simulink model "HEVPlant_Ptbs_V1b_MkSfunc"  (R2018b)
settings: configuration reference "Config_Plant_MkSfunc_FIxStep" (kept outside this file)
PreLoadFcn:
  | HEVPlant_Ptbs_V1_BusInfo
model workspace (MAT data in the model file):
  DiffRatio = 3.421
  EV_current = 200
  EV_motion = [20 4 0.8]
  EV_sf = 2000
  EngDriveRatio = 0.813008130081
  Fs = 0
  Fv = 0.0025
  Jcomp = 0.0227
  Jengine = 0.22
  Ki = 251.3274
  Kisa = 346.6583
  Kp_d = 0.47149
  Kp_q = 0.52125
  Ksa = 85.4316
  Ksf = 1996.2651
  Ld = 0.0003752
  Ldq = [0.0003752 0.0004148]
  Lq = 0.0004148
  Mechanical = [0.0227 0.0025 0]
  MotGbRatio = 1
  P = 4
  PolePairs = 4
  RWheel = 0.3
  Rs = 0.2
  T_max = 120
  T_mtpa = [0 13.3131834767 26.6278836885 39.9456159322 53.2678926341 66.5962219318 79.9321062746 93.277041051 106.632513247 120.000000141]
  MCOS : class17 (value not decoded)
  MCOS : class17 (value not decoded)
  ba = 3.4029
  id_mtpa = [0 -0.114523352646 -0.457989076459 -1.03008464374 -1.83029075221 -2.85788367342 -4.11193850568 -5.59133329791 -7.29475400168 -9.22070020138]
  idq0 = [0 0]
  idq_limits = [-9.220699542 166.993501392 167.247872355]
  iq_mtpa = [0 18.5827440345 37.1633719111 55.7397734896 74.3098506185 92.871523015 111.422734008 129.961456105 148.485696337 166.993501356]
  MCOS : class17 (value not decoded)
  MCOS : class17 (value not decoded)
  lambda_pm = 0.1194
  mechanical = [0.0227 0.0025 0]
  mot : struct (value not decoded)
  omega_init = 0
  theta_init = 0
  MCOS : class17 (value not decoded)
symbols that are objects in the model workspace (value not decoded): mot
libraries: autolibshared x4, autolibsharedcoupling x2, autolibtransamt x1, autolibshareddiff x1, autolibsharedmappedengines x1, simulink x1, autolibdatasheetbattery x1, autolibmappedmotor x1
(part 5 of 5)

== system HEVPlant_Ptbs_V1b_MkSfunc/Engine/Info_in ==
  Bus Creator1 : BusCreator  Inputs=1
  Constant : Constant
  Info_in : Outport
  wires:
  Constant/1 -> Bus Creator1/1  "dummy"
  Bus Creator1/1 -> Info_in/1  "Info_in"

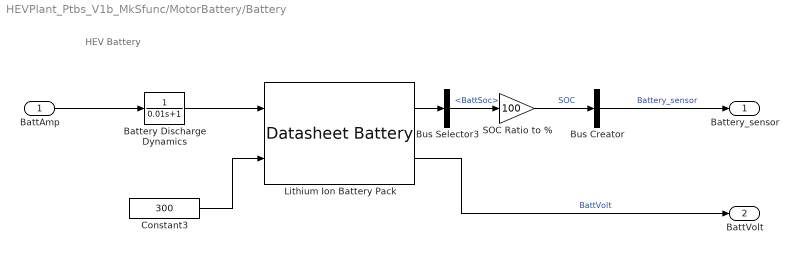
== system HEVPlant_Ptbs_V1b_MkSfunc/MotorBattery/Battery ==
  note: HEV Battery
  BattAmp : Inport
  Battery Discharge Dynamics : TransferFcn  Denominator=[0.01 1]
  Bus Creator : BusCreator  Inputs=1  OutDataTypeStr=Bus: Battery_sensor_Bus
      settings: AttributesFormatString=%<OutDataTypeStr>
  Bus Selector3 : BusSelector  OutputSignals=BattSoc
  Constant3 : Constant  Value=300
  Lithium Ion Battery Pack : autolibdatasheetbattery/Datasheet Battery  CapacityCtrl=Parameter  OutputVlt=Unfiltered  BattChargeMax=7  Em=[2.8 3.228 3.284 3.361 3.408 3.427 3.472 3.477 3.493 3.504 3.516 3.528 3.537 3.545 3.555 3.561 3.566 3.576 3.587 3.589 3.594 3.6 3.608 3.61 3.616 3.619 3.626 3.632 3.637 3.64 3.645 3.646 3.652 3.655 3.658 3.661 3.664 3.668 3.673 3.678 3.68 3.681 3.686 3.692 3.699 3.702 3.705 3.71 3.717 3.723 3.728 3.733 3.735 3.742 3.749 3.755 3.761 3.768 3.773 3.78 3.791 3.798 3.798 3.814 3.818 3.825 3.841 3.846 3.855 3.863 3.877 3.885 3.894 3.907 3.919 3.926 3.935 3.944 3.954 3.964 3.974 3.988 3.998 4.014 4.029 4.034 4.047 4.065 4.074 4.086 4.097 4.131 4.126 4.138 4.15 4.18 4.174 4.187 4.207 4.231 4.221]  CapLUTBp=[0 0.01 0.02 0.03 0.04 0.05 0.06 0.07 0.08 0.09 0.1 0.11 0.12 0.13 0.14 0.15 0.16 0.17 0.18 0.19 0.2 0.21 0.22 0.23 0.24 0.25 0.26 0.27 0.28 0.29 0.3 0.31 0.32 0.33 0.34 0.35 0.36 0.37 0.38 0.39 0.4 0.41 0.42 0.43 0.44 0.45 0.46 0.47 0.48 0.49 0.5 0.51 0.52 0.53 0.54 0.55 0.56 0.57 0.58 0.59 0.6 0.61 0.62 0.63 0.64 0.65 0.66 0.67 0.68 0.69 0.7 0.71 0.72 0.73 0.74 0.75 0.76 0.77 0.78 0.79 0.8 0.81 0.82 0.83 0.84 0.85 0.86 0.87 0.88 0.89 0.9 0.91 0.92 0.93 0.94 0.95 0.96 0.97 0.98 0.99 1]  RInt=[0.008846 0.009319 0.009027 0.00847 0.01032 0.01314;0.006389 0.006554 0.005553 0.005525 0.006043 0.007805;0.004364 0.004101 0.00406 0.003452 0.003846 0.004517;0.002031 0.002563 0.002532 0.00246 0.002716 0.003047;0.001443 0.001825 0.001795 0.001778 0.001924 0.002234;0.0005603 0.0007192 0.0006887 0.0007557 0.0007355 0.001014;0.001028 0.001338 0.001 0.001536 0.001546 0.002789]  BattTempBp=[243.1 253.1 263.1 273.1 283.1 298.1 313.1]  CapSOCBp=[0 0.2 0.4 0.6 0.8 1]  Ns=320/4.2  Np=1  BattCapInit=7*.6  Tc=1/1000  Vinit=4.221
      settings: SourceProductName=Powertrain Blockset  SourceProductBaseCode=PW
  SOC Ratio to % : Gain  Gain=100
  Battery_sensor : Outport
  BattVolt : Outport  Port=2
  wires:
  SOC Ratio to %/1 -> Bus Creator/1  "SOC"
  Lithium Ion Battery Pack/1 -> Bus Selector3/1
  Bus Selector3/1 -> SOC Ratio to %/1  "<BattSoc>"
  Constant3/1 -> Lithium Ion Battery Pack/2
  Battery Discharge Dynamics/1 -> Lithium Ion Battery Pack/1
  Bus Creator/1 -> Battery_sensor/1  "Battery_sensor"
  Lithium Ion Battery Pack/2 -> BattVolt/1  "BattVolt"
  BattAmp/1 -> Battery Discharge Dynamics/1

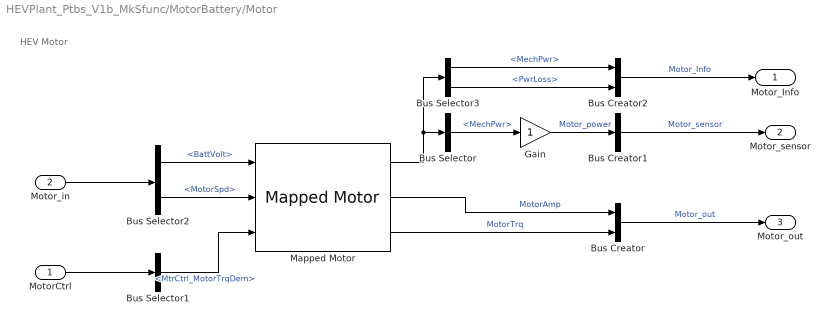
== system HEVPlant_Ptbs_V1b_MkSfunc/MotorBattery/Motor ==
  note: HEV Motor
  MotorCtrl : Inport  OutDataTypeStr=Bus: MotorCtrl_Bus  SampleTime=0
      settings: AttributesFormatString=%<OutDataTypeStr>
  Motor_in : Inport  Port=2  OutDataTypeStr=Bus: Motor_in_Bus
      settings: AttributesFormatString=%<OutDataTypeStr>
  Bus Creator : BusCreator  Inputs=2  OutDataTypeStr=Bus: Motor_out_Bus
      settings: AttributesFormatString=%<OutDataTypeStr>
  Bus Creator1 : BusCreator  Inputs=1  OutDataTypeStr=Bus: Motor_sensor_Bus
      settings: AttributesFormatString=%<OutDataTypeStr>
  Bus Creator2 : BusCreator  Inputs=2  OutDataTypeStr=Bus: Motor_Info_out_Bus
      settings: AttributesFormatString=%<OutDataTypeStr>
  Bus Selector : BusSelector  OutputSignals=MechPwr
  Bus Selector1 : BusSelector  OutputSignals=MtrCtrl_MotorTrqDem
  Bus Selector2 : BusSelector  OutputSignals=BattVolt,MotorSpd
  Bus Selector3 : BusSelector  OutputSignals=MechPwr,PwrLoss
  Gain : Gain
  Mapped Motor : autolibmappedmotor/Mapped Motor  port_config=Speed  param_by=Maximum torque and power  w_t=[ 0 375 750 800 ]  T_t=[0.09 0.08 0.07 0]  torque_max=307  power_max=124e3  Tc=0.02  param_loss=Tabulated efficiency data  eff=100  w_eff=375  T_eff=0.08  Piron=0  Pbase=0  w_eff_bp=mot.map.spdindex.*pi/30  T_eff_bp=mot.map.trqindex  losses_table=[1 2;3 4]  efficiency_table=mot.map.eff'  J=5e-6  b=1e-5  omega_o=0  T_t_extended=[0 0.07 0.08 0.09 0.08 0.07 0]  w_t_extended=[-800 -750 -375 0 375 750 800]  KLossIron=0  KLossCopper=0  x_w_eff_vec=[-1317.7933984258 -1256.63706143592 -1151.91730631626 -1047.1975511966 -942.477796076938 -837.758040957278 -733.038285837618 -628.318530717959 -523.598775598299 -418.879020478639 -403.904095496528 -314.159265358979 -209.43951023932 -104.71975511966 0 104.71975511966 209.43951023932 314.159265358979 403.904095496528 418.879020478639 523.598775598299 628.318530717959 733.038285837618 837.758040957278 942.477796076938 1047.1975511966 1151.91730631626 1256.63706143592 1317.7933984258]  x_T_eff_vec=[-307 -300 -275 -250 -225 -200 -175 -150 -125 -100 -75 -50 -25 -10 10 25 50 75 100 125 150 175 200 225 250 275 300 307]  x_losses_mat=[44951.3970351912 43926.4466141933 40265.9093963439 36605.3721784944 32944.834960645 29284.2977427955 25623.7605249461 21963.2233070967 18302.6860892472 14642.1488713978 7439.15628143595 4959.4375209573 2479.71876047865 1464.21488713978 1317.7933984258 2306.13844724515 4612.27689449029 6918.41534173544 13177.933984258 16472.4174803225 19766.900976387 23061.3844724515 26355.867968516 29650.3514645805 32944.834960645 36239.3184567095 39533.801952774 40456.257331672;29037.7746776966 28375.675580811 26011.0359490768 23646.3963173425 21281.7566856083 18917.117053874 16552.4774221398 14187.8377904055 11823.1981586713 9458.558526937 7093.91889520275 4729.2792634685 2364.63963173425 1396.26340159546 1256.63706143592 2199.11485751285 4398.22971502571 6597.34457253856 8796.45943005141 10995.5742875643 13194.6891450771 15393.80400259 17592.9188601028 19792.0337176157 21991.1485751285 24190.2634326414 26389.3782901542 27005.1304502578;26617.9601212219 26011.0359490768 23843.449619987 21675.8632908973 19508.2769618076 17340.6906327178 15173.1043036281 13005.5179745384 10837.9316454486 8670.34531635892 4547.0419986168 3031.3613324112 2167.58632908973 1279.90811812918 1151.91730631626 2015.85528605345 2879.79326579064 4319.68989868596 8063.4211442138 10079.2764302672 12095.1317163207 14110.9870023741 16126.8422884276 18142.697574481 20158.5528605345 22174.4081465879 24190.2634326414 24754.7029127364;24198.1455647472 23646.3963173425 21675.8632908973 19705.3302644521 17734.7972380069 15764.2642115617 13793.7311851165 11823.1981586713 9852.66513222605 7882.13210578084 4133.67454419709 2755.78302946473 1970.53302644521 1163.55283466289 1047.1975511966 1832.59571459404 2617.99387799149 3926.99081698724 7330.38285837618 9162.97857297022 10995.5742875643 12828.1700021583 14660.7657167524 16493.3614313464 18325.9571459404 20158.5528605345 21991.1485751285 22504.2753752149;21778.3310082725 21281.7566856083 19508.2769618076 17734.7972380069 15961.3175142062 14187.8377904055 12414.3580666048 10640.8783428041 6200.51181629564 4960.40945303651 3720.30708977738 2480.20472651826 1240.10236325913 1047.1975511966 942.477796076938 1178.09724509617 2356.19449019234 3534.29173528851 4712.38898038468 5890.48622548085 9896.01685880784 11545.3530019425 13194.6891450771 14844.0252882118 16493.3614313464 18142.697574481 19792.0337176157 20253.8478376934;19358.5164517977 18917.117053874 17340.6906327178 15764.2642115617 14187.8377904055 12611.4113692493 11034.9849480932 9458.558526937 5511.56605892945 4409.25284714356 3306.93963535767 2204.62642357178 1102.31321178589 930.842267730309 837.758040957278 1047.1975511966 2094.39510239319 3141.59265358979 4188.79020478639 5235.98775598298 8796.45943005141 10262.5360017266 11728.6125734019 13194.6891450771 14660.7657167524 16126.8422884276 17592.9188601028 18003.4203001719;16938.701895323 16552.4774221398 15173.1043036281 13793.7311851165 12414.3580666048 11034.9849480932 9655.61182958152 5787.14436187593 4822.62030156327 3054.32619099008 2290.74464324256 1527.16309549504 964.524060312655 814.486984264021 733.038285837618 916.297857297022 1466.07657167524 2199.11485751286 2932.15314335048 4581.48928648511 5497.78714378213 8979.71900151082 10262.5360017266 11545.3530019425 12828.1700021583 14110.9870023741 15393.80400259 15752.9927626504;14518.8873388483 14187.8377904055 13005.5179745384 11823.1981586713 10640.8783428041 9458.558526937 8276.23871106988 4960.40945303651 3272.49234748937 2617.9938779915 1963.49540849362 1653.46981767884 826.734908839418 698.131700797732 628.318530717959 785.398163397447 1570.79632679489 1884.95559215388 2513.27412287184 3141.5926535898 4712.38898038468 7696.90200129499 8796.45943005141 9896.01685880784 10995.5742875643 12095.1317163207 13194.6891450771 13502.5652251289;17860.5360120753 17453.2925199433 15998.8514766147 14544.4104332861 13089.9693899575 7882.13210578084 6896.86559255823 4133.67454419709 3444.72878683091 2181.66156499292 1636.24617374469 1090.83078249646 545.415391248229 ...(+9284 chars)]  aMode=aMode
      settings: SourceProductName=Powertrain Blockset  SourceProductBaseCode=PW
  Motor_Info : Outport  OutDataTypeStr=Bus: Motor_Info_out_Bus
      settings: AttributesFormatString=%<OutDataTypeStr>
  Motor_sensor : Outport  Port=2  OutDataTypeStr=Bus: Motor_sensor_Bus
      settings: AttributesFormatString=%<OutDataTypeStr>
  Motor_out : Outport  Port=3  OutDataTypeStr=Bus: Motor_out_Bus
      settings: AttributesFormatString=%<OutDataTypeStr>
  wires:
  Bus Selector2/2 -> Mapped Motor/2  "<MotorSpd>"
  Mapped Motor/1 -> Bus Selector3/1, Bus Selector/1
  Bus Selector2/1 -> Mapped Motor/1  "<BattVolt>"
  Mapped Motor/3 -> Bus Creator/2  "MotorTrq"
  Bus Selector1/1 -> Mapped Motor/3  "<MtrCtrl_MotorTrqDem>"
  Bus Creator1/1 -> Motor_sensor/1  "Motor_sensor"
  Motor_in/1 -> Bus Selector2/1
  Gain/1 -> Bus Creator1/1  "Motor_power"
  Bus Selector/1 -> Gain/1  "<MechPwr>"
  Mapped Motor/2 -> Bus Creator/1  "MotorAmp"
  Bus Selector3/1 -> Bus Creator2/1  "<MechPwr>"
  MotorCtrl/1 -> Bus Selector1/1
  Bus Creator/1 -> Motor_out/1  "Motor_out"
  Bus Selector3/2 -> Bus Creator2/2  "<PwrLoss>"
  Bus Creator2/1 -> Motor_Info/1  "Motor_Info"

== system HEVPlant_Ptbs_V1b_MkSfunc/Engine/Engine/Engine Sensor ==
  Info : Inport
  Bus Creator : BusCreator  Inputs=2  OutDataTypeStr=Bus: Engine_sensor_Bus
      settings: AttributesFormatString=%<OutDataTypeStr>
  Bus Selector3 : BusSelector  OutputSignals=EngSpd,CrkAng
  Gain : Gain
  Signal Specification : SignalSpecification
  Engine_sensor : Outport
  wires:
  Gain/1 -> Bus Creator/1  "EngineSpd"
  Bus Creator/1 -> Engine_sensor/1  "Engine_sensor"
  Info/1 -> Bus Selector3/1
  Bus Selector3/2 -> Signal Specification/1  "<CrkAng>"
  Bus Selector3/1 -> Gain/1  "<EngSpd>"
  Signal Specification/1 -> Bus Creator/2  "CrankAngle"

== system HEVPlant_Ptbs_V1b_MkSfunc/Engine/Engine/Info ==
  Info : Inport
  Bus Creator1 : BusCreator  Inputs=2  OutDataTypeStr=Bus: Eng_Info_out_Bus
      settings: AttributesFormatString=%<OutDataTypeStr>
  Bus Selector5 : BusSelector  OutputSignals=FuelMassFlw,EngSpd
  Eng_Info_out : Outport
  wires:
  Bus Creator1/1 -> Eng_Info_out/1  "Eng_Info_out"
  Info/1 -> Bus Selector5/1
  Bus Selector5/2 -> Bus Creator1/2  "<EngSpd>"
  Bus Selector5/1 -> Bus Creator1/1  "<FuelMassFlw>"
